simulink model "oqpsk_syn"  (Simulink 7.9)
settings: Solver=FixedStepDiscrete  SolverMode=SingleTasking  StartTime=0.0  StopTime=1e2  RelTol=1e-3
PreLoadFcn:
  | oqpsk_syn_init;
undefined symbols (not defined in the file or in its folder): get, oqpsk_syn_params, rcosfir
libraries: shlslibv1 x26, commsink2 x6, commutil2 x2, commchan3 x1, commrandsrc2 x1, dspsigops x1
settings Model: synDspstartup=OK  Creator=sszilvasi  LastModifiedBy=sszilvasi
settings DataIOCC: SaveOutput=off  SignalLogging=off  SaveTime=off
settings OptimizationCC: InlineParams=on
settings DebuggingCC: AlgebraicLoopMsg=error  InheritedTsInSrcMsg=none

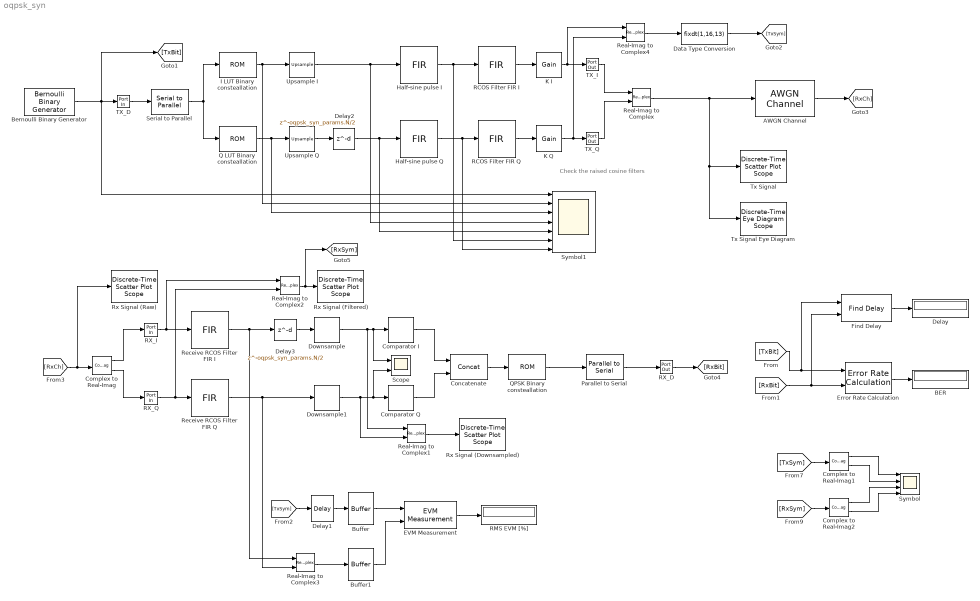
== system oqpsk_syn ==
  note: Check the raised cosine filters
  AWGN Channel : commchan3/AWGN Channel  InputProcessing=Columns as channels (frame based)  seed=67  noiseMode="Signal to noise ratio  (SNR)"  EbNodB=30  EsNodB=10  SNRdB=oqpsk_syn_params.snr  bitsPerSym=1  Ps=1  Tsym=1  variance=1
  BER : Display
  Bernoulli Binary Generator : commrandsrc2/Bernoulli Binary Generator  P=0.5  seed=61  Ts=1  frameBased=off  sampPerFrame=1  orient=off  outDataType=double
  Buffer : Buffer  TreatMby1Signals=One channel
  Buffer1 : Buffer  TreatMby1Signals=One channel
  Comparator I : shlslibv1/Math Functions/Comparator  syn_comp_opr=a>b  syn_comp_const=on  syn_comp_val=0  synBlockType=primitive  synLatency=0  synBlockId=14
  Comparator Q : shlslibv1/Math Functions/Comparator  syn_comp_opr=a>b  syn_comp_const=on  syn_comp_val=0  synBlockType=primitive  synLatency=0  synBlockId=14
  Complex to Real-Imag : ComplexToRealImag
  Complex to Real-Imag1 : ComplexToRealImag
  Complex to Real-Imag2 : ComplexToRealImag
  Concatenate : shlslibv1/Signal Operations/Concat  syn_in_nb=2  syn_out_f=Automatic  syn_out_wl=16  syn_out_fl=8  syn_out_dt=signed  synBlockType=primitive  synLatency=0  synBlockId=8
  Data Type Conversion : DataTypeConversion  OutDataTypeStr=fixdt(1,16,13)
  Delay : Display
  Delay1 : dspsigops/Delay  InputProcessing=Columns as channels (frame based)  dly_unit=Samples  delay=8  ic_detail=off  dif_ic_for_ch=off  dif_ic_for_dly=off  ic=0  reset_popup=None
  Delay2 : Delay  DelayLength=oqpsk_syn_params.N/2
  Delay3 : Delay  DelayLength=oqpsk_syn_params.N/2
  Downsample : shlslibv1/Signal Operations/Downsample  syn_r_val=oqpsk_syn_params.N  syn_sample_offset=8  syn_sync_mode=No Sync  synBlockType=primitive  synLatency=1  synBlockId=7
  Downsample1 : shlslibv1/Signal Operations/Downsample  syn_r_val=oqpsk_syn_params.N  syn_sample_offset=8  syn_sync_mode=No Sync  synBlockType=primitive  synLatency=1  synBlockId=7
  EVM Measurement : commutil2/EVM Measurement  normMethod=Average reference signal power  averagePower=1  peakPower=1  maxOrMinOut=off  percentileOut=off  percentileVal=95  nSym=off
  Error Rate Calculation : commsink2/Error Rate Calculation  N=14  st_delay=0  cp_mode=Entire frame  subframe=[]  PMode=Port  WsName=ErrorVec  RsMode2=off  stop=off  numErr=100  maxBits=1e6
  Find Delay : commutil2/Find Delay  corrLength=200  chgSigOP=off  stopUpdate=off  numConstDelay=3
  Half-sine pulse I : shlslibv1/Filtering/FIR  syn_coef_vec=sin(pi/oqpsk_syn_params.N*[0:oqpsk_syn_params.N-1])  syn_coef_fl=15  syn_coef_rnd=Nearest  syn_show_q=off  syn_dp_f=Automatic  syn_dp_wl=16  syn_dp_fl=8  syn_dp_sat=off  syn_dp_rnd=Floor (Truncate)  syn_out_f=Specify  syn_out_wl=16  syn_out_fl=13  syn_out_dt=signed  syn_out_sat=off  syn_out_rnd=Floor (Truncate)  syn_rst_port=off  syn_en_port=off  synBlockType=primitive  synLatency=0  synBlockId=80
  Half-sine pulse Q : shlslibv1/Filtering/FIR  syn_coef_vec=sin(pi/oqpsk_syn_params.N*[0:oqpsk_syn_params.N-1])  syn_coef_fl=15  syn_coef_rnd=Nearest  syn_show_q=off  syn_dp_f=Automatic  syn_dp_wl=16  syn_dp_fl=8  syn_dp_sat=off  syn_dp_rnd=Floor (Truncate)  syn_out_f=Specify  syn_out_wl=16  syn_out_fl=13  syn_out_dt=signed  syn_out_sat=off  syn_out_rnd=Floor (Truncate)  syn_rst_port=off  syn_en_port=off  synBlockType=primitive  synLatency=0  synBlockId=80
  "I LUT Binary consteallation " : shlslibv1/Memories/ROM  syn_rom_vec=[1 -1 -1 1]  syn_out_wl=2  syn_out_fl=0  syn_out_dt=signed  syn_out_sat=off  syn_out_rnd=on  synBlockType=primitive  synLatency=1  synBlockId=62
  K I : shlslibv1/Math Functions/Gain  syn_gain_val=1/2  syn_gain_fl=2  syn_gain_dt=signed  syn_gain_rnd=on  syn_out_f=Full Precision  syn_out_wl=16  syn_out_fl=8  syn_out_dt=signed  syn_out_sat=off  syn_out_rnd=Floor (Truncate)  synBlockType=primitive  synLatency=0  synBlockId=3  syn_opr_mode=0
  K Q : shlslibv1/Math Functions/Gain  syn_gain_val=1/2  syn_gain_fl=2  syn_gain_dt=signed  syn_gain_rnd=on  syn_out_f=Full Precision  syn_out_wl=16  syn_out_fl=8  syn_out_dt=signed  syn_out_sat=off  syn_out_rnd=Floor (Truncate)  synBlockType=primitive  synLatency=0  synBlockId=3  syn_opr_mode=0
  Parallel to Serial : shlslibv1/Signal Operations/Parallel to Serial  syn_pack_nb=2  syn_pack_ord=LSB to MSB  synBlockType=custom  synLatency=0
  Q LUT Binary consteallation : shlslibv1/Memories/ROM  syn_rom_vec=[1 1 -1 -1]  syn_out_wl=2  syn_out_fl=0  syn_out_dt=signed  syn_out_sat=off  syn_out_rnd=on  synBlockType=primitive  synLatency=1  synBlockId=62
  QPSK Binary consteallation : shlslibv1/Memories/ROM  syn_rom_vec=[2 1 3 0]  syn_out_wl=2  syn_out_fl=0  syn_out_dt=unsigned  syn_out_sat=off  syn_out_rnd=on  synBlockType=primitive  synLatency=1  synBlockId=62
  RCOS Filter FIR I : shlslibv1/Filtering/FIR  syn_coef_vec=rcosfir(0.5,5,4,1,'sqrt')  syn_coef_fl=15  syn_coef_rnd=Nearest  syn_show_q=off  syn_dp_f=Automatic  syn_dp_wl=16  syn_dp_fl=8  syn_dp_sat=off  syn_dp_rnd=Floor (Truncate)  syn_out_f=Specify  syn_out_wl=16  syn_out_fl=13  syn_out_dt=signed  syn_out_sat=off  syn_out_rnd=Floor (Truncate)  syn_rst_port=off  syn_en_port=off  synBlockType=primitive  synLatency=0  synBlockId=80
  RCOS Filter FIR Q : shlslibv1/Filtering/FIR  syn_coef_vec=rcosfir(0.5,5,4,1,'sqrt')  syn_coef_fl=15  syn_coef_rnd=Nearest  syn_show_q=off  syn_dp_f=Automatic  syn_dp_wl=16  syn_dp_fl=8  syn_dp_sat=off  syn_dp_rnd=Floor (Truncate)  syn_out_f=Specify  syn_out_wl=16  syn_out_fl=13  syn_out_dt=signed  syn_out_sat=off  syn_out_rnd=Floor (Truncate)  syn_rst_port=off  syn_en_port=off  synBlockType=primitive  synLatency=0  synBlockId=80
  RMS EVM [%] : Display
  RX_D : shlslibv1/Ports & Subsystems/Port Out  syn_capture=off  syn_register=off  synBlockType=port  synLatency=0  synBlockId=1
  RX_I : shlslibv1/Ports & Subsystems/Port In  syn_out_wl=16  syn_out_fl=14  syn_out_dt=signed  syn_out_st=-1  syn_capture=off  syn_register=off  syn_out_sat=off  syn_out_rnd=on  synBlockType=port  synLatency=0  synBlockId=0
  RX_Q : shlslibv1/Ports & Subsystems/Port In  syn_out_wl=16  syn_out_fl=14  syn_out_dt=signed  syn_out_st=-1  syn_capture=off  syn_register=off  syn_out_sat=off  syn_out_rnd=on  synBlockType=port  synLatency=0  synBlockId=0
  Real-Imag to Complex{,1..4} (5 alike) : RealImagToComplex
  Receive RCOS Filter FIR I : shlslibv1/Filtering/FIR  syn_coef_vec=rcosfir(0.5,5,4,1,'sqrt')  syn_coef_fl=15  syn_coef_rnd=Nearest  syn_show_q=off  syn_dp_f=Automatic  syn_dp_wl=16  syn_dp_fl=8  syn_dp_sat=off  syn_dp_rnd=Floor (Truncate)  syn_out_f=Specify  syn_out_wl=16  syn_out_fl=13  syn_out_dt=signed  syn_out_sat=off  syn_out_rnd=Floor (Truncate)  syn_rst_port=off  syn_en_port=off  synBlockType=primitive  synLatency=0  synBlockId=80
  Receive RCOS Filter FIR Q : shlslibv1/Filtering/FIR  syn_coef_vec=rcosfir(0.5,5,4,1,'sqrt')  syn_coef_fl=15  syn_coef_rnd=Nearest  syn_show_q=off  syn_dp_f=Automatic  syn_dp_wl=16  syn_dp_fl=8  syn_dp_sat=off  syn_dp_rnd=Floor (Truncate)  syn_out_f=Specify  syn_out_wl=16  syn_out_fl=13  syn_out_dt=signed  syn_out_sat=off  syn_out_rnd=Floor (Truncate)  syn_rst_port=off  syn_en_port=off  synBlockType=primitive  synLatency=0  synBlockId=80
  Rx Signal (Downsampled) : commsink2/Discrete-Time Scatter Plot Scope  Tag=ScatterPlot  sampPerSymb=1  offsetEye=0  numTraces=200  numNewFrames=40  LineMarkers=.  LineColors=b  fading=on  render=on  AxisGrid=on  xMin=-2.2368896484375  xMax=2.36206420898437  yMin=-2.29389785766602  yMax=2.30505599975586  inphaseLabel=In-phase Amplitude  quadratureLabel=Quadrature Amplitude  openScopeAtSimStart=off  FrameNumber=off  FigPos=get(0,'defaultfigureposition');  figTitle=Scatter Plot  numLinesMax=8  block_type_=scatter
  Rx Signal (Filtered) : commsink2/Discrete-Time Scatter Plot Scope  Tag=ScatterPlot  sampPerSymb=oqpsk_syn_params.N  offsetEye=12  numTraces=200  numNewFrames=40  LineMarkers=.  LineColors=b  fading=on  render=on  AxisGrid=on  xMin=-3.36879364013672  xMax=3.36598480224609  yMin=-3.36634521484375  yMax=3.36843322753906  inphaseLabel=In-phase Amplitude  quadratureLabel=Quadrature Amplitude  openScopeAtSimStart=off  FrameNumber=off  FigPos=get(0,'defaultfigureposition');  figTitle=Scatter Plot  numLinesMax=8  block_type_=scatter
  Rx Signal (Raw) : commsink2/Discrete-Time Scatter Plot Scope  Tag=ScatterPlot  sampPerSymb=oqpsk_syn_params.N  offsetEye=8  numTraces=200  numNewFrames=40  LineMarkers=.  LineColors=b  fading=on  render=on  AxisGrid=on  xMin=-2.21685054225205  xMax=2.21272506884322  yMin=-2.21171497145292  yMax=2.21786063964235  inphaseLabel=In-phase Amplitude  quadratureLabel=Quadrature Amplitude  openScopeAtSimStart=off  FrameNumber=off  FigPos=get(0,'defaultfigureposition');  figTitle=Scatter Plot  numLinesMax=8  block_type_=scatter
  Scope : Scope  NumInputPorts=2
      settings: YMin=-5~-5  YMax=5~5
  Serial to Parallel : shlslibv1/Signal Operations/Serial to Parallel  syn_pack_nb=2  syn_pack_ord=LSB to MSB  syn_out_f=Automatic  syn_out_wl=17  syn_out_fl=9  syn_out_dt=signed  synBlockType=custom  synLatency=1
  Symbol : Scope  NumInputPorts=4
      settings: YMin=-5~-5~-5~-5  YMax=5~5~5~5  SaveName=ScopeData3
  Symbol1 : Scope  NumInputPorts=7
      settings: YMin=-5~-5~-5~-5~-5~-5~-5  YMax=5~5~5~5~5~5~5
  TX_D : shlslibv1/Ports & Subsystems/Port In  syn_out_wl=1  syn_out_fl=0  syn_out_dt=unsigned  syn_out_st=-1  syn_capture=off  syn_register=off  syn_out_sat=off  syn_out_rnd=on  synBlockType=port  synLatency=0  synBlockId=0
  TX_I : shlslibv1/Ports & Subsystems/Port Out  syn_capture=off  syn_register=off  synBlockType=port  synLatency=0  synBlockId=1
  TX_Q : shlslibv1/Ports & Subsystems/Port Out  syn_capture=off  syn_register=off  synBlockType=port  synLatency=0  synBlockId=1
  Tx Signal : commsink2/Discrete-Time Scatter Plot Scope  Tag=ScatterPlot  sampPerSymb=oqpsk_syn_params.N  offsetEye=8  numTraces=200  numNewFrames=40  LineMarkers=.  LineColors=b  fading=on  render=on  AxisGrid=on  xMin=-2.21417953491211  xMax=2.2104899597168  yMin=-2.20969848632812  yMax=2.21497100830078  inphaseLabel=In-phase Amplitude  quadratureLabel=Quadrature Amplitude  openScopeAtSimStart=off  FrameNumber=off  FigPos=get(0,'defaultfigureposition');  figTitle=Scatter Plot  numLinesMax=8  block_type_=scatter
  Tx Signal Eye Diagram : commsink2/Discrete-Time Eye Diagram Scope  Tag=EyeDiagram  sampPerSymb=8  offsetEye=0  symbPerTrace=1  numTraces=40  numNewFrames=10  LineStyles=-  LineColors=b  dupPoints=on  fading=on  render=on  AxisGrid=on  yMin=-18.129248046875  yMax=6.77067138671875  inphaseLabel=In-phase Amplitude  quadratureLabel=Quadrature Amplitude  openScopeAtSimStart=off  dispDiagram=In-phase and Quadrature  FrameNumber=off  FigPos=get(0,'defaultfigureposition');  figTitle=Eye Diagram  block_type_=eye  numLinesMax=8
  Upsample I : shlslibv1/Signal Operations/Upsample  syn_r_val=oqpsk_syn_params.N  syn_in_hold=off  syn_sample_offset=0  syn_sync_mode=No Sync  synBlockType=primitive  synLatency=0  synBlockId=6
  Upsample Q : shlslibv1/Signal Operations/Upsample  syn_r_val=oqpsk_syn_params.N  syn_in_hold=off  syn_sample_offset=0  syn_sync_mode=No Sync  synBlockType=primitive  synLatency=0  synBlockId=6
  wires:
  [TxBit] -> Error Rate Calculation/1, Find Delay/1
  [RxBit] -> Error Rate Calculation/2, Find Delay/2
  Error Rate Calculation/1 -> BER/1
  EVM Measurement/1 -> RMS EVM [%]/1
  Buffer1/1 -> EVM Measurement/2
  [TxSym] -> Delay1/1
  Delay1/1 -> Buffer/1
  Buffer/1 -> EVM Measurement/1
  Upsample Q/1 -> Delay2/1
  TX_D/1 -> Serial to Parallel/1
  Q LUT Binary consteallation/1 -> Upsample Q/1, Symbol1/3
  RCOS Filter FIR Q/1 -> K Q/1
  TX_I/1 -> Real-Imag to Complex/1
  TX_Q/1 -> Real-Imag to Complex/2
  K Q/1 -> TX_Q/1, Real-Imag to Complex4/2
  Real-Imag to Complex/1 -> AWGN Channel/1, Tx Signal/1, Tx Signal Eye Diagram/1
  RCOS Filter FIR I/1 -> K I/1
  K I/1 -> TX_I/1, Real-Imag to Complex4/1
  "I LUT Binary consteallation "/1 -> Upsample I/1, Symbol1/2
  Serial to Parallel/1 -> Q LUT Binary consteallation/1, "I LUT Binary consteallation "/1
  Bernoulli Binary Generator/1 -> TX_D/1, [TxBit], Symbol1/1
  [RxCh] -> Complex to Real-Imag/1, Rx Signal (Raw)/1
  Complex to Real-Imag/1 -> RX_I/1
  Complex to Real-Imag/2 -> RX_Q/1
  AWGN Channel/1 -> [RxCh]
  RX_I/1 -> Receive RCOS Filter FIR I/1, Real-Imag to Complex2/1
  RX_Q/1 -> Receive RCOS Filter FIR Q/1, Real-Imag to Complex2/2
  Receive RCOS Filter FIR I/1 -> Real-Imag to Complex3/1, Delay3/1
  Receive RCOS Filter FIR Q/1 -> Real-Imag to Complex3/2, Downsample1/1
  Parallel to Serial/1 -> RX_D/1
  RX_D/1 -> [RxBit]
  Downsample/1 -> Real-Imag to Complex1/1, Comparator I/1, Scope/1
  Downsample1/1 -> Real-Imag to Complex1/2, Comparator Q/1, Scope/2
  Real-Imag to Complex1/1 -> Rx Signal (Downsampled)/1
  Concatenate/1 -> QPSK Binary consteallation/1
  Real-Imag to Complex2/1 -> Rx Signal (Filtered)/1, [RxSym]
  Real-Imag to Complex3/1 -> Buffer1/1
  Real-Imag to Complex4/1 -> Data Type Conversion/1
  [TxSym] -> Complex to Real-Imag1/1
  [RxSym] -> Complex to Real-Imag2/1
  Complex to Real-Imag1/1 -> Symbol/1
  Complex to Real-Imag1/2 -> Symbol/2
  Complex to Real-Imag2/1 -> Symbol/3
  Complex to Real-Imag2/2 -> Symbol/4
  Comparator I/1 -> Concatenate/1
  Comparator Q/1 -> Concatenate/2
  QPSK Binary consteallation/1 -> Parallel to Serial/1
  Find Delay/1 -> Delay/1
  Upsample I/1 -> Half-sine pulse I/1, Symbol1/4
  Half-sine pulse I/1 -> RCOS Filter FIR I/1, Symbol1/6
  Delay2/1 -> Half-sine pulse Q/1, Symbol1/5
  Half-sine pulse Q/1 -> RCOS Filter FIR Q/1, Symbol1/7
  Delay3/1 -> Downsample/1
  Data Type Conversion/1 -> [TxSym]
